simulink model "ejercicio1"  (R2024a)
settings: Solver=VariableStepAuto  StartTime=0.0  StopTime=10.0  RelTol=1e-3
settings Model: Creator=pablo  LastModifiedBy=pablo

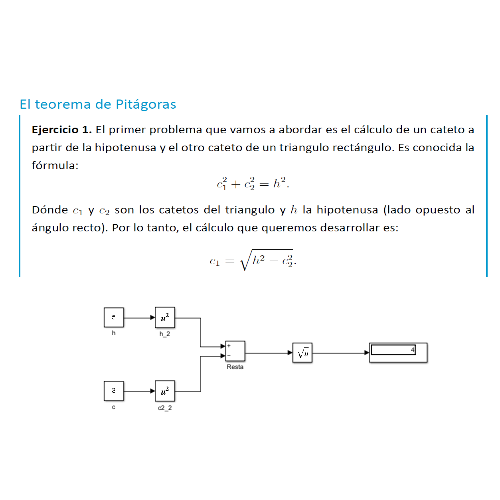
[thumbnail: Simulink's stored preview of the top-level diagram]
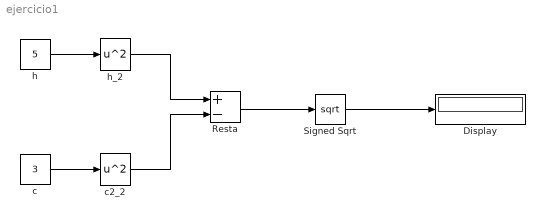
== system ejercicio1 ==
  Display : Display
  Resta : Sum  Inputs=+-
  Signed Sqrt : Sqrt
  c : Constant  Value=3
  c2_2 : Math  Operator=square
  h : Constant  Value=5
  h_2 : Math  Operator=square
  wires:
  h/1 -> h_2/1
  c/1 -> c2_2/1
  h_2/1 -> Resta/1
  c2_2/1 -> Resta/2
  Resta/1 -> Signed Sqrt/1
  Signed Sqrt/1 -> Display/1
